simulink model "car_ctrl_V"  (R2021a)
settings: Solver=VariableStepAuto  StartTime=0.0  StopTime=inf  RelTol=1e-3
undefined symbols (not defined in the file or in its folder): cal_P
libraries: simulink x2
settings Model: Creator=think  LastModifiedBy=ASUS
settings SolverCC: AlgebraicLoopSolver=TrustRegion
settings DataIOCC: ReturnWorkspaceOutputs=off
settings DebuggingCC: SFMachineParentedDataDiag=warning  ArithmeticOperatorsInVariantConditions=warning
settings SFSimCC: SimUseLocalCustomCode=off  CustomCodeUndefinedFunction=UseInterfaceOnly
settings RTWCC: RTWUseLocalCustomCode=off
settings CodeAppCC: StateflowObjectComments=on

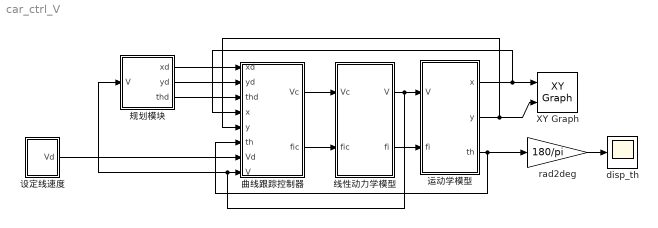
== system car_ctrl_V ==
  XY Graph : simulink/Sinks/XY Graph  xmin=-3  xmax=3  ymin=-0.2  ymax=5.2  st=-1
  disp_th : Scope
  rad2deg : Gain  Gain=180/pi
  曲线跟踪控制器 : Subsystem
  线性动力学模型 : Subsystem  mask{Tv=0.1, Tfi=0.1}
      mask prompts: Tv "小车速度驱动时间常数(秒)"; Tfi "小车转向驱动时间常数(秒)"
  规划模块 : Subsystem
  设定线速度 : Subsystem
  运动学模型 : Subsystem  mask{L=0.254}
      mask prompts: L "小车车长Ｌ(米)"
  wires:
  线性动力学模型/1(V) -> 规划模块/1(V), 曲线跟踪控制器/8(V), 运动学模型/1(V)
  运动学模型/3(th) -> rad2deg/1, 曲线跟踪控制器/6(th)
  rad2deg/1 -> disp_th/1
  运动学模型/1(x) -> XY Graph/1, 曲线跟踪控制器/4(x)
  运动学模型/2(y) -> 曲线跟踪控制器/5(y), XY Graph/2
  曲线跟踪控制器/1(Vc) -> 线性动力学模型/1(Vc)
  曲线跟踪控制器/2(fic) -> 线性动力学模型/2(fic)
  线性动力学模型/2(fi) -> 运动学模型/2(fi)
  规划模块/1(xd) -> 曲线跟踪控制器/1(xd)
  规划模块/2(yd) -> 曲线跟踪控制器/2(yd)
  规划模块/3(thd) -> 曲线跟踪控制器/3(thd)
  设定线速度/1(Vd) -> 曲线跟踪控制器/7(Vd)

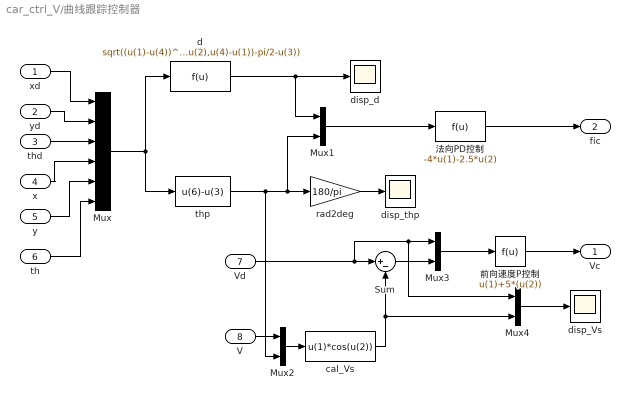
== system car_ctrl_V/曲线跟踪控制器 ==
  xd : Inport
  yd : Inport  Port=2
  thd : Inport  Port=3
  x : Inport  Port=4
  y : Inport  Port=5
  th : Inport  Port=6
  Vd : Inport  Port=7
  V : Inport  Port=8
  Mux : Mux  Inputs=6
  Mux{1..4} (4 alike) : Mux  Inputs=2
  Sum : Sum  Inputs=|+-
  cal_Vs : Fcn  Expr=u(1)*cos(u(2))
  d : Fcn  Expr=sqrt((u(1)-u(4))^2+(u(2)-u(5))^2)*cos(atan2(u(5)-u(2),u(4)-u(1))-pi/2-u(3))
  disp_Vs : Scope
  disp_d : Scope
  disp_thp : Scope
  rad2deg : Gain  Gain=180/pi
  thp : Fcn  Expr=u(6)-u(3)
  前向速度P控制 : Fcn  Expr=u(1)+5*(u(2))
  法向PD控制 : Fcn  Expr=-4*u(1)-2.5*u(2)
  Vc : Outport
  fic : Outport  Port=2
  wires:
  th/1 -> Mux/6
  xd/1 -> Mux/1
  x/1 -> Mux/4
  thd/1 -> Mux/3
  前向速度P控制/1 -> Vc/1
  y/1 -> Mux/5
  法向PD控制/1 -> fic/1
  yd/1 -> Mux/2
  Mux/1 -> d/1, thp/1
  d/1 -> disp_d/1, Mux1/1
  Mux1/1 -> 法向PD控制/1
  thp/1 -> rad2deg/1, Mux1/2, Mux2/2
  rad2deg/1 -> disp_thp/1
  Vd/1 -> Mux4/1, Mux3/1, Sum/1
  V/1 -> Mux2/1
  Mux2/1 -> cal_Vs/1
  cal_Vs/1 -> Mux4/2, Sum/2
  Sum/1 -> Mux3/2
  Mux3/1 -> 前向速度P控制/1
  Mux4/1 -> disp_Vs/1

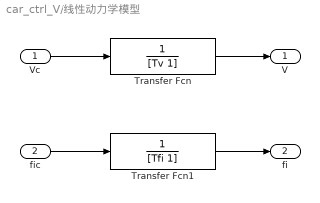
== system car_ctrl_V/线性动力学模型 ==
  Vc : Inport
  fic : Inport  Port=2
  Transfer Fcn : TransferFcn  Denominator=[Tv 1]
  Transfer Fcn1 : TransferFcn  Denominator=[Tfi 1]
  V : Outport
  fi : Outport  Port=2
  wires:
  Vc/1 -> Transfer Fcn/1
  fic/1 -> Transfer Fcn1/1
  Transfer Fcn1/1 -> fi/1
  Transfer Fcn/1 -> V/1

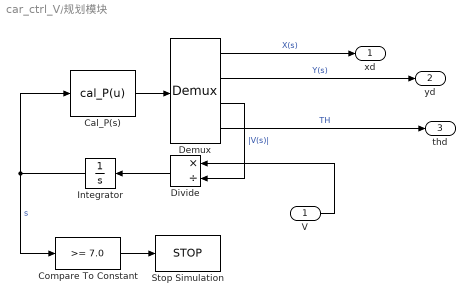
== system car_ctrl_V/规划模块 ==
  V : Inport
  Cal_P(s) : MATLABFcn  MATLABFcn=cal_P(u)  OutputDimensions=4
  Compare To Constant : simulink/Logic and Bit Operations/Compare To Constant  relop=>=  const=7.0  OutDataTypeStr=boolean  ZeroCross=off
  Demux : Demux
  Divide : Product  Inputs=*/
  Integrator : Integrator
  Stop Simulation : Stop
  xd : Outport
  yd : Outport  Port=2
  thd : Outport  Port=3
  wires:
  Cal_P(s)/1 -> Demux/1
  V/1 -> Divide/1
  Compare To Constant/1 -> Stop Simulation/1
  Divide/1 -> Integrator/1
  Integrator/1 -> Cal_P(s)/1, Compare To Constant/1  "s"
  Demux/1 -> xd/1  "X(s)"
  Demux/2 -> yd/1  "Y(s)"
  Demux/3 -> Divide/2  "|V(s)|"
  Demux/4 -> thd/1  "TH"

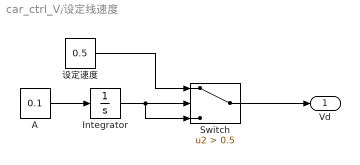
== system car_ctrl_V/设定线速度 ==
  A : Constant  Value=0.1
  Integrator : Integrator
  Switch : Switch  Criteria=u2 > Threshold  Threshold=0.5
  设定速度 : Constant  Value=0.5
  Vd : Outport
  wires:
  Switch/1 -> Vd/1
  Integrator/1 -> Switch/3, Switch/2
  A/1 -> Integrator/1
  设定速度/1 -> Switch/1

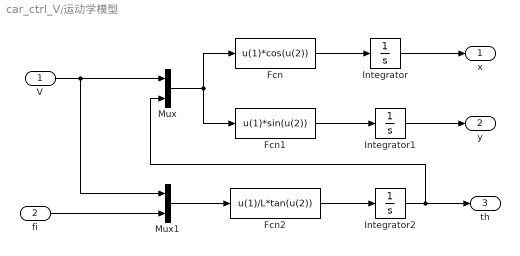
== system car_ctrl_V/运动学模型 ==
  V : Inport
  fi : Inport  Port=2
  Fcn : Fcn  Expr=u(1)*cos(u(2))
  Fcn1 : Fcn  Expr=u(1)*sin(u(2))
  Fcn2 : Fcn  Expr=u(1)/L*tan(u(2))
  Integrator : Integrator
  Integrator1 : Integrator
  Integrator2 : Integrator
  Mux : Mux  Inputs=2
  Mux1 : Mux  Inputs=2
  x : Outport
  y : Outport  Port=2
  th : Outport  Port=3
  wires:
  Mux/1 -> Fcn1/1, Fcn/1
  Fcn/1 -> Integrator/1
  Fcn2/1 -> Integrator2/1
  Mux1/1 -> Fcn2/1
  Integrator2/1 -> th/1, Mux/2
  V/1 -> Mux1/1, Mux/1
  Integrator/1 -> x/1
  Integrator1/1 -> y/1
  fi/1 -> Mux1/2
  Fcn1/1 -> Integrator1/1
